simulink model "problem__9"  (R2020a)
settings: Solver=VariableStepAuto  StartTime=0.0  StopTime=10.0  RelTol=1e-3
undefined symbols (not defined in the file): B, J, K, L, P, R
settings Model: Creator=USER  LastModifiedBy=USER

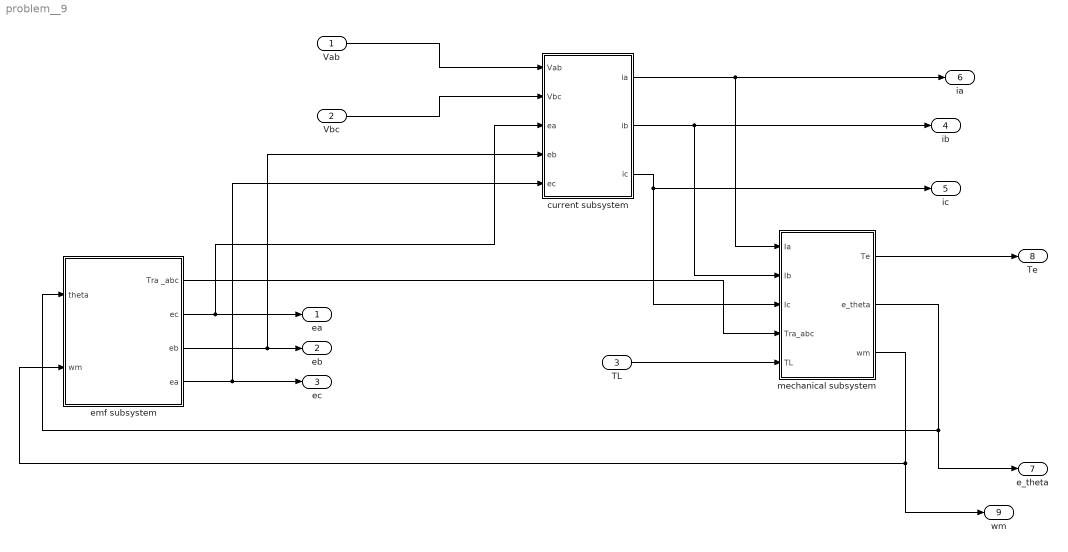
== system problem__9 ==
  Vab : Inport
  Vbc : Inport  Port=2
  TL : Inport  Port=3
  current subsystem : Subsystem
  emf subsystem : Subsystem
  mechanical subsystem : Subsystem
  ea : Outport
  eb : Outport  Port=2
  ec : Outport  Port=3
  ib : Outport  Port=4
  ic : Outport  Port=5
  ia : Outport  Port=6
  e_theta : Outport  Port=7
  Te : Outport  Port=8
  wm : Outport  Port=9
  wires:
  emf subsystem/4(ea) -> ec/1, current subsystem/5(ec)
  emf subsystem/2(ec) -> ea/1, current subsystem/3(ea)
  mechanical subsystem/1(Te) -> Te/1
  mechanical subsystem/2(e_theta) -> e_theta/1, emf subsystem/1(theta)
  TL/1 -> mechanical subsystem/5(TL)
  current subsystem/3(ic) -> ic/1, mechanical subsystem/3(Ic)
  mechanical subsystem/3(wm) -> wm/1, emf subsystem/2(wm)
  emf subsystem/3(eb) -> eb/1, current subsystem/4(eb)
  current subsystem/1(ia) -> ia/1, mechanical subsystem/1(Ia)
  Vab/1 -> current subsystem/1(Vab)
  current subsystem/2(ib) -> ib/1, mechanical subsystem/2(Ib)
  Vbc/1 -> current subsystem/2(Vbc)
  emf subsystem/1(Tra _abc) -> mechanical subsystem/4(Tra_abc)

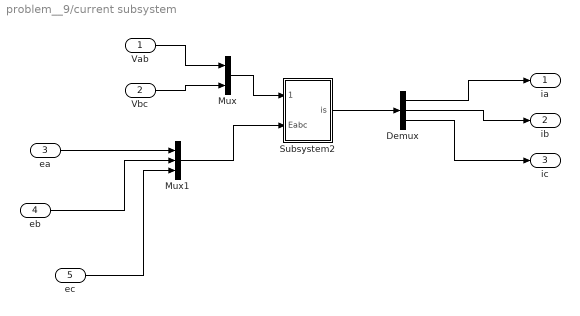
== system problem__9/current subsystem ==
  Vab : Inport
  Vbc : Inport  Port=2
  ea : Inport  Port=3
  eb : Inport  Port=4
  ec : Inport  Port=5
  Demux : Demux  Outputs=3
  Mux : Mux  Inputs=2
  Mux1 : Mux  Inputs=3
  Subsystem2 : Subsystem
  ia : Outport
  ib : Outport  Port=2
  ic : Outport  Port=3
  wires:
  ea/1 -> Mux1/1
  Vbc/1 -> Mux/2
  Demux/3 -> ic/1
  Subsystem2/1(is) -> Demux/1
  eb/1 -> Mux1/2
  Demux/2 -> ib/1
  ec/1 -> Mux1/3
  Demux/1 -> ia/1
  Vab/1 -> Mux/1
  Mux1/1 -> Subsystem2/2(Eabc)
  Mux/1 -> Subsystem2/1(Vab,Vbc)

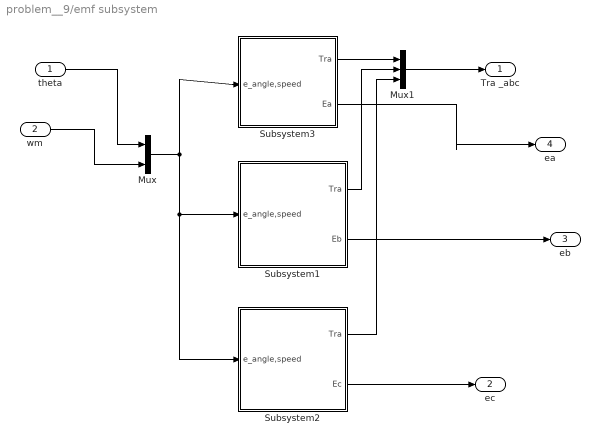
== system problem__9/emf subsystem ==
  theta : Inport
  wm : Inport  Port=2
  Mux : Mux  Inputs=2
  Mux1 : Mux  Inputs=3
  Subsystem1 : Subsystem
  Subsystem2 : Subsystem
  Subsystem3 : Subsystem
  Tra _abc : Outport
  ec : Outport  Port=2
  eb : Outport  Port=3
  ea : Outport  Port=4
  wires:
  Subsystem3/2(Ea) -> ea/1
  Mux/1 -> Subsystem1/1(e_angle,speed), Subsystem2/1(e_angle,speed), Subsystem3/1(e_angle,speed)
  theta/1 -> Mux/1
  Subsystem2/2(Ec) -> ec/1
  Subsystem1/1(Tra) -> Mux1/2
  Subsystem3/1(Tra) -> Mux1/1
  Subsystem1/2(Eb) -> eb/1
  Subsystem2/1(Tra) -> Mux1/3
  wm/1 -> Mux/2
  Mux1/1 -> Tra _abc/1

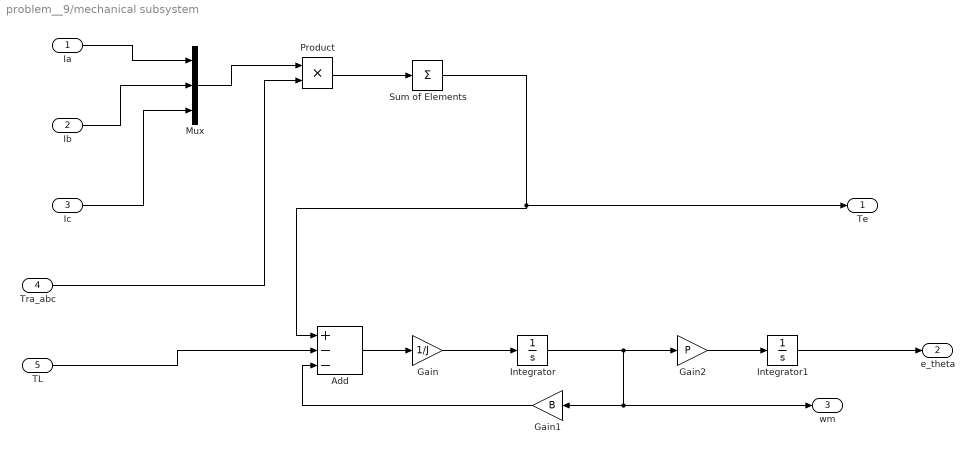
== system problem__9/mechanical subsystem ==
  Ia : Inport
  Ib : Inport  Port=2
  Ic : Inport  Port=3
  Tra_abc : Inport  Port=4
  TL : Inport  Port=5
  Add : Sum  Inputs=+--
  Gain : Gain  Gain=1/J
  Gain1 : Gain  Gain=B
  Gain2 : Gain  Gain=P
  Integrator : Integrator
  Integrator1 : Integrator
  Mux : Mux  Inputs=3
  Product : Product
  Sum of Elements : Sum  Inputs=+
  Te : Outport
  e_theta : Outport  Port=2
  wm : Outport  Port=3
  wires:
  Tra_abc/1 -> Product/2
  Sum of Elements/1 -> Te/1, Add/1
  Gain2/1 -> Integrator1/1
  Integrator/1 -> Gain2/1, wm/1, Gain1/1
  Ib/1 -> Mux/2
  Product/1 -> Sum of Elements/1
  Add/1 -> Gain/1
  Mux/1 -> Product/1
  Integrator1/1 -> e_theta/1
  TL/1 -> Add/2
  Gain1/1 -> Add/3
  Ia/1 -> Mux/1
  Gain/1 -> Integrator/1
  Ic/1 -> Mux/3

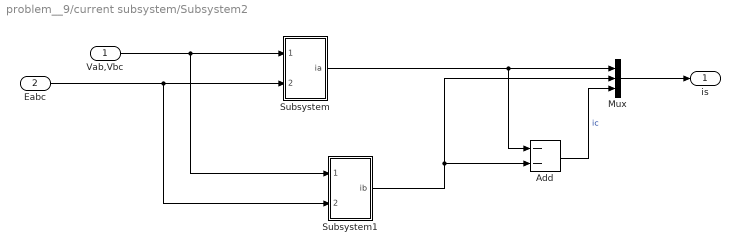
== system problem__9/current subsystem/Subsystem2 ==
  Vab,Vbc : Inport
  Eabc : Inport  Port=2
  Add : Sum  Inputs=--
  Mux : Mux  Inputs=3
  Subsystem : Subsystem
  Subsystem1 : Subsystem
  is : Outport
  wires:
  Mux/1 -> is/1
  Subsystem1/1(ib) -> Add/2, Mux/2
  Vab,Vbc/1 -> Subsystem1/1(Vab,Vbc), Subsystem/1(Vab,Vbc)
  Eabc/1 -> Subsystem1/2(Eabc), Subsystem/2(Eabc)
  Subsystem/1(ia) -> Add/1, Mux/1
  Add/1 -> Mux/3  "ic"

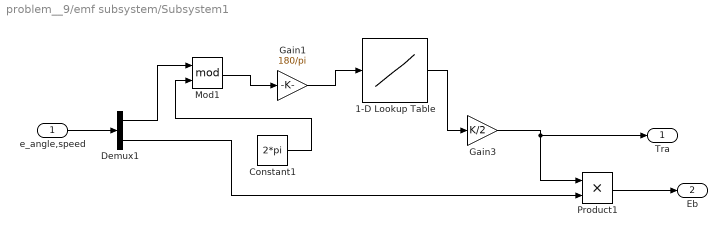
== system problem__9/emf subsystem/Subsystem1 ==
  e_angle,speed : Inport
  1-D Lookup Table : Lookup_n-D  NumberOfTableDimensions=1  BreakpointsForDimension1=[0,40,60,120,180,240,300,320,360]  Table=[-1,-1,-1,1,1,1,-1,-1,-1]  InterpMethod=Cubic spline  InternalRulePriority=Speed  RndMeth=Simplest  InputSameDT=on
  Constant1 : Constant  Value=2*pi
  Demux1 : Demux  Outputs=2
  Gain1 : Gain  Gain=180/pi
  Gain3 : Gain  Gain=K/2
  Mod1 : Math  Operator=mod  SaturateOnIntegerOverflow=on
  Product1 : Product
  Tra : Outport
  Eb : Outport  Port=2
  wires:
  Gain3/1 -> Tra/1, Product1/1
  Demux1/1 -> Mod1/1
  e_angle,speed/1 -> Demux1/1
  Constant1/1 -> Mod1/2
  Demux1/2 -> Product1/2
  Mod1/1 -> Gain1/1
  Product1/1 -> Eb/1
  Gain1/1 -> 1-D Lookup Table/1
  1-D Lookup Table/1 -> Gain3/1

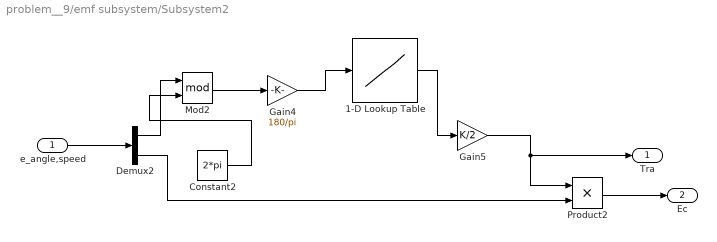
== system problem__9/emf subsystem/Subsystem2 ==
  e_angle,speed : Inport
  1-D Lookup Table : Lookup_n-D  NumberOfTableDimensions=1  BreakpointsForDimension1=[0,60,80,120,180,240,275,360]  Table=[1,-1,-1,-1,-1,1,1,1]  InterpMethod=Cubic spline  InternalRulePriority=Speed  RndMeth=Simplest  InputSameDT=on
  Constant2 : Constant  Value=2*pi
  Demux2 : Demux  Outputs=2
  Gain4 : Gain  Gain=180/pi
  Gain5 : Gain  Gain=K/2
  Mod2 : Math  Operator=mod  SaturateOnIntegerOverflow=on
  Product2 : Product
  Tra : Outport
  Ec : Outport  Port=2
  wires:
  e_angle,speed/1 -> Demux2/1
  Demux2/2 -> Product2/2
  Gain5/1 -> Tra/1, Product2/1
  Constant2/1 -> Mod2/2
  Demux2/1 -> Mod2/1
  Product2/1 -> Ec/1
  Mod2/1 -> Gain4/1
  Gain4/1 -> 1-D Lookup Table/1
  1-D Lookup Table/1 -> Gain5/1

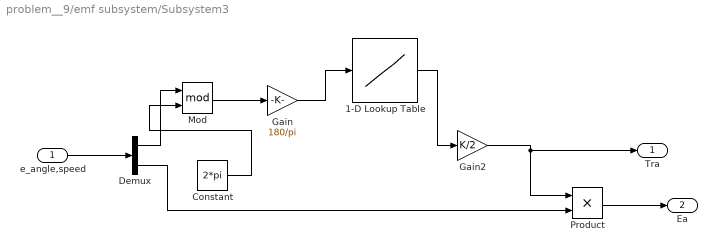
== system problem__9/emf subsystem/Subsystem3 ==
  e_angle,speed : Inport
  1-D Lookup Table : Lookup_n-D  NumberOfTableDimensions=1  BreakpointsForDimension1=[0,40,60,80,120,180,250,275,300,360]  Table=[1,1,1,1,1,-1,-1,-1,-1,1]  InterpMethod=Cubic spline  InternalRulePriority=Speed  RndMeth=Simplest  InputSameDT=on
  Constant : Constant  Value=2*pi
  Demux : Demux  Outputs=2
  Gain : Gain  Gain=180/pi
  Gain2 : Gain  Gain=K/2
  Mod : Math  Operator=mod  SaturateOnIntegerOverflow=on
  Product : Product
  Tra : Outport
  Ea : Outport  Port=2
  wires:
  Product/1 -> Ea/1
  Mod/1 -> Gain/1
  Demux/2 -> Product/2
  Gain2/1 -> Tra/1, Product/1
  Gain/1 -> 1-D Lookup Table/1
  Demux/1 -> Mod/1
  e_angle,speed/1 -> Demux/1
  Constant/1 -> Mod/2
  1-D Lookup Table/1 -> Gain2/1

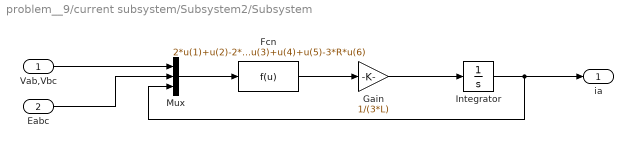
== system problem__9/current subsystem/Subsystem2/Subsystem ==
  Vab,Vbc : Inport
  Eabc : Inport  Port=2
  Fcn : Fcn  Expr=2*u(1)+u(2)-2*u(3)+u(4)+u(5)-3*R*u(6)
  Gain : Gain  Gain=1/(3*L)
  Integrator : Integrator
  Mux : Mux  Inputs=3
  ia : Outport
  wires:
  Integrator/1 -> ia/1, Mux/3
  Gain/1 -> Integrator/1
  Vab,Vbc/1 -> Mux/1
  Mux/1 -> Fcn/1
  Fcn/1 -> Gain/1
  Eabc/1 -> Mux/2

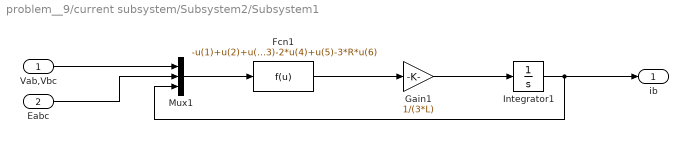
== system problem__9/current subsystem/Subsystem2/Subsystem1 ==
  Vab,Vbc : Inport
  Eabc : Inport  Port=2
  Fcn1 : Fcn  Expr=-u(1)+u(2)+u(3)-2*u(4)+u(5)-3*R*u(6)
  Gain1 : Gain  Gain=1/(3*L)
  Integrator1 : Integrator
  Mux1 : Mux  Inputs=3
  ib : Outport
  wires:
  Integrator1/1 -> ib/1, Mux1/3
  Fcn1/1 -> Gain1/1
  Gain1/1 -> Integrator1/1
  Vab,Vbc/1 -> Mux1/1
  Eabc/1 -> Mux1/2
  Mux1/1 -> Fcn1/1
